simulink library "UXFD_Lib"  (R2016b)
settings: Solver=ode45  StartTime=0.0  StopTime=10.0  RelTol=1e-3  EnableMultiTasking=on
undefined symbols (not defined in the file): BreakpointData, BreakpointData1, BreakpointData2, BreakpointData_One_A, BreakpointData_Two_A, E2E_P01DataIDMode, E2E_P01ReceiverStatusType, EnumClass, iBit, initalValue, No_Runnable_Period, ObB_EidBsgStDerat_C, p_OVERRIDE_MASTER_SWITCH, SlDemoSign, SwitchOff_P, SwitchOn_P, Table, TableData_M, VCCTi33, VSysD_FidVehDerat1_C
libraries: simulink x28, CCMLib x11, UXFD_Lib x8, canmsglib x2, PTCC_Lib x1, hdlsllib x1
(part 6 of 7)

== system UXFD_Lib/Standard/Discrete dynamics/LPF2_omega ==
  u : Inport
  w : Inport  Port=2
  z : Inport  Port=3
  Constant : Constant  Value=2  mask(TL_Constant){data={'output',{'type','Float32'},'date',735300.29222866893}}
      settings: CopyFcn=if exist('tl_reset_reviewflag','file')==2,tl_reset_reviewflag(gcbh);end  DeleteFcn=if exist('delete_tlblock','file')==2,delete_tlblock(gcbh);end  NameChangeFcn=if exist('rename_tlblock','file')==2,rename_tlblock(gcbh);end  OpenFcn=if exist('tl_open_blockdlg','file')==2,tl_open_blockdlg(gcbh);else,open_system(gcbh,'parameter');end
      mask Help: eval(['if exist(''tl_online_help'',''file'') == 2, tl_online_help(''Topic'',''TL_Constant''),else, web([''jar:file:///'',matlabroot,''/help/toolbox/simulink/help.jar!/slref/' lower(get_param(gcbh,'Blocktype')) '.html''], ''-helpbrowser''),end'])
      mask Display: plot([-0.05, 1.05, NaN, -0.05, 1.05],[.01, .01, NaN, .99, .99])
  Constant2 : Constant  Value=2  mask(TL_Constant){data={'output',{'type','Float32'},'date',735300.29222841433}}
      settings: CopyFcn=if exist('tl_reset_reviewflag','file')==2,tl_reset_reviewflag(gcbh);end  DeleteFcn=if exist('delete_tlblock','file')==2,delete_tlblock(gcbh);end  NameChangeFcn=if exist('rename_tlblock','file')==2,rename_tlblock(gcbh);end  OpenFcn=if exist('tl_open_blockdlg','file')==2,tl_open_blockdlg(gcbh);else,open_system(gcbh,'parameter');end
      mask Help: eval(['if exist(''tl_online_help'',''file'') == 2, tl_online_help(''Topic'',''TL_Constant''),else, web([''jar:file:///'',matlabroot,''/help/toolbox/simulink/help.jar!/slref/' lower(get_param(gcbh,'Blocktype')) '.html''], ''-helpbrowser''),end'])
      mask Display: plot([-0.05, 1.05, NaN, -0.05, 1.05],[.01, .01, NaN, .99, .99])
  Constant3 : Constant  mask(TL_Constant){data={'output',{'type','Float32'},'date',735300.29222815973}}
      settings: CopyFcn=if exist('tl_reset_reviewflag','file')==2,tl_reset_reviewflag(gcbh);end  DeleteFcn=if exist('delete_tlblock','file')==2,delete_tlblock(gcbh);end  NameChangeFcn=if exist('rename_tlblock','file')==2,rename_tlblock(gcbh);end  OpenFcn=if exist('tl_open_blockdlg','file')==2,tl_open_blockdlg(gcbh);else,open_system(gcbh,'parameter');end
      mask Help: eval(['if exist(''tl_online_help'',''file'') == 2, tl_online_help(''Topic'',''TL_Constant''),else, web([''jar:file:///'',matlabroot,''/help/toolbox/simulink/help.jar!/slref/' lower(get_param(gcbh,'Blocktype')) '.html''], ''-helpbrowser''),end'])
      mask Display: plot([-0.05, 1.05, NaN, -0.05, 1.05],[.01, .01, NaN, .99, .99])
  Product : Product  Inputs=**  SaturateOnIntegerOverflow=on  RndMeth=Zero  InputSameDT=on  OutDataTypeStr=Inherit: Same as first input  mask(TL_Product){data={'logdata',{'maxnumvals',4096,'plotchannels',[]},'output',{'type','Float32'},'date',735300.29222787032}}
      settings: CopyFcn=if exist('tl_reset_reviewflag','file')==2,tl_reset_reviewflag(gcbh);end  DeleteFcn=if exist('delete_tlblock','file')==2,delete_tlblock(gcbh);end  NameChangeFcn=if exist('rename_tlblock','file')==2,rename_tlblock(gcbh);end  OpenFcn=if exist('tl_open_blockdlg','file')==2,tl_open_blockdlg(gcbh);else,open_system(gcbh,'parameter');end
      mask Help: eval(['if exist(''tl_online_help'',''file'') == 2, tl_online_help(''Topic'',''TL_Product''),else, web([''jar:file:///'',matlabroot,''/help/toolbox/simulink/help.jar!/slref/' lower(get_param(gcbh,'Blocktype')) '.html''], ''-helpbrowser''),end'])
      mask Display: plot([-0.05, 1.05, NaN, -0.05, 1.05],[.01, .01, NaN, .99, .99])
  Product1 : Product  Inputs=***  SaturateOnIntegerOverflow=on  RndMeth=Zero  InputSameDT=on  OutDataTypeStr=Inherit: Same as first input  mask(TL_Product){data={'logdata',{'maxnumvals',4096,'plotchannels',[]},'output',{'type','Float32'},'date',735300.29222759255}}
      settings: CopyFcn=if exist('tl_reset_reviewflag','file')==2,tl_reset_reviewflag(gcbh);end  DeleteFcn=if exist('delete_tlblock','file')==2,delete_tlblock(gcbh);end  NameChangeFcn=if exist('rename_tlblock','file')==2,rename_tlblock(gcbh);end  OpenFcn=if exist('tl_open_blockdlg','file')==2,tl_open_blockdlg(gcbh);else,open_system(gcbh,'parameter');end
      mask Help: eval(['if exist(''tl_online_help'',''file'') == 2, tl_online_help(''Topic'',''TL_Product''),else, web([''jar:file:///'',matlabroot,''/help/toolbox/simulink/help.jar!/slref/' lower(get_param(gcbh,'Blocktype')) '.html''], ''-helpbrowser''),end'])
      mask Display: plot([-0.05, 1.05, NaN, -0.05, 1.05],[.01, .01, NaN, .99, .99])
  Product3 : Product  Inputs=**  SaturateOnIntegerOverflow=on  RndMeth=Zero  InputSameDT=on  OutDataTypeStr=Inherit: Same as first input  mask(TL_Product){data={'logdata',{'maxnumvals',4096,'plotchannels',[]},'output',{'type','Float32'},'date',735300.29222732643}}
      settings: CopyFcn=if exist('tl_reset_reviewflag','file')==2,tl_reset_reviewflag(gcbh);end  DeleteFcn=if exist('delete_tlblock','file')==2,delete_tlblock(gcbh);end  NameChangeFcn=if exist('rename_tlblock','file')==2,rename_tlblock(gcbh);end  OpenFcn=if exist('tl_open_blockdlg','file')==2,tl_open_blockdlg(gcbh);else,open_system(gcbh,'parameter');end
      mask Help: eval(['if exist(''tl_online_help'',''file'') == 2, tl_online_help(''Topic'',''TL_Product''),else, web([''jar:file:///'',matlabroot,''/help/toolbox/simulink/help.jar!/slref/' lower(get_param(gcbh,'Blocktype')) '.html''], ''-helpbrowser''),end'])
      mask Display: plot([-0.05, 1.05, NaN, -0.05, 1.05],[.01, .01, NaN, .99, .99])
  Product4 : Product  Inputs=**  SaturateOnIntegerOverflow=on  RndMeth=Zero  InputSameDT=on  OutDataTypeStr=Inherit: Same as first input  mask(TL_Product){data={'logdata',{'maxnumvals',4096,'plotchannels',[]},'output',{'type','Float32'},'date',735300.29222704866}}
      settings: CopyFcn=if exist('tl_reset_reviewflag','file')==2,tl_reset_reviewflag(gcbh);end  DeleteFcn=if exist('delete_tlblock','file')==2,delete_tlblock(gcbh);end  NameChangeFcn=if exist('rename_tlblock','file')==2,rename_tlblock(gcbh);end  OpenFcn=if exist('tl_open_blockdlg','file')==2,tl_open_blockdlg(gcbh);else,open_system(gcbh,'parameter');end
      mask Help: eval(['if exist(''tl_online_help'',''file'') == 2, tl_online_help(''Topic'',''TL_Product''),else, web([''jar:file:///'',matlabroot,''/help/toolbox/simulink/help.jar!/slref/' lower(get_param(gcbh,'Blocktype')) '.html''], ''-helpbrowser''),end'])
      mask Display: plot([-0.05, 1.05, NaN, -0.05, 1.05],[.01, .01, NaN, .99, .99])
  Product5 : Product  Inputs=*/  SaturateOnIntegerOverflow=on  RndMeth=Zero  InputSameDT=on  OutDataTypeStr=Inherit: Same as first input  mask(TL_Product){data={'logdata',{'maxnumvals',4096,'plotchannels',[]},'output',{'type','Float32'},'date',735300.29222677078}}
      settings: CopyFcn=if exist('tl_reset_reviewflag','file')==2,tl_reset_reviewflag(gcbh);end  DeleteFcn=if exist('delete_tlblock','file')==2,delete_tlblock(gcbh);end  NameChangeFcn=if exist('rename_tlblock','file')==2,rename_tlblock(gcbh);end  OpenFcn=if exist('tl_open_blockdlg','file')==2,tl_open_blockdlg(gcbh);else,open_system(gcbh,'parameter');end
      mask Help: eval(['if exist(''tl_online_help'',''file'') == 2, tl_online_help(''Topic'',''TL_Product''),else, web([''jar:file:///'',matlabroot,''/help/toolbox/simulink/help.jar!/slref/' lower(get_param(gcbh,'Blocktype')) '.html''], ''-helpbrowser''),end'])
      mask Display: plot([-0.05, 1.05, NaN, -0.05, 1.05],[.01, .01, NaN, .99, .99])
  Product6 : Product  Inputs=**  SaturateOnIntegerOverflow=on  RndMeth=Zero  InputSameDT=on  OutDataTypeStr=Inherit: Same as first input  mask(TL_Product){data={'logdata',{'maxnumvals',4096,'plotchannels',[]},'output',{'type','Float32'},'date',735300.29222649301}}
      settings: CopyFcn=if exist('tl_reset_reviewflag','file')==2,tl_reset_reviewflag(gcbh);end  DeleteFcn=if exist('delete_tlblock','file')==2,delete_tlblock(gcbh);end  NameChangeFcn=if exist('rename_tlblock','file')==2,rename_tlblock(gcbh);end  OpenFcn=if exist('tl_open_blockdlg','file')==2,tl_open_blockdlg(gcbh);else,open_system(gcbh,'parameter');end
      mask Help: eval(['if exist(''tl_online_help'',''file'') == 2, tl_online_help(''Topic'',''TL_Product''),else, web([''jar:file:///'',matlabroot,''/help/toolbox/simulink/help.jar!/slref/' lower(get_param(gcbh,'Blocktype')) '.html''], ''-helpbrowser''),end'])
      mask Display: plot([-0.05, 1.05, NaN, -0.05, 1.05],[.01, .01, NaN, .99, .99])
  Sum1 : Sum  Inputs=+--  SaturateOnIntegerOverflow=on  InputSameDT=on  OutDataTypeStr=Inherit: Same as first input  mask(TL_Sum){data={'logdata',{'maxnumvals',4096,'plotchannels',[]},'output',{'type','Float32'},'date',735300.29222619208}}
      settings: CopyFcn=if exist('tl_reset_reviewflag','file')==2,tl_reset_reviewflag(gcbh);end  DeleteFcn=if exist('delete_tlblock','file')==2,delete_tlblock(gcbh);end  NameChangeFcn=if exist('rename_tlblock','file')==2,rename_tlblock(gcbh);end  OpenFcn=if exist('tl_open_blockdlg','file')==2,tl_open_blockdlg(gcbh);else,open_system(gcbh,'parameter');end
      mask Help: eval(['if exist(''tl_online_help'',''file'') == 2, tl_online_help(''Topic'',''TL_Sum''),else, web([''jar:file:///'',matlabroot,''/help/toolbox/simulink/help.jar!/slref/' lower(get_param(gcbh,'Blocktype')) '.html''], ''-helpbrowser''),end'])
      mask Display: plot([-0.05, 1.05, NaN, -0.05, 1.05],[.01, .01, NaN, .99, .99])
  Sum2 : Sum  Inputs=--  SaturateOnIntegerOverflow=on  InputSameDT=on  OutDataTypeStr=Inherit: Same as first input  mask(TL_Sum){data={'logdata',{'maxnumvals',4096,'plotchannels',[]},'output',{'type','Float32'},'date',735300.29222592595}}
      settings: CopyFcn=if exist('tl_reset_reviewflag','file')==2,tl_reset_reviewflag(gcbh);end  DeleteFcn=if exist('delete_tlblock','file')==2,delete_tlblock(gcbh);end  NameChangeFcn=if exist('rename_tlblock','file')==2,rename_tlblock(gcbh);end  OpenFcn=if exist('tl_open_blockdlg','file')==2,tl_open_blockdlg(gcbh);else,open_system(gcbh,'parameter');end
      mask Help: eval(['if exist(''tl_online_help'',''file'') == 2, tl_online_help(''Topic'',''TL_Sum''),else, web([''jar:file:///'',matlabroot,''/help/toolbox/simulink/help.jar!/slref/' lower(get_param(gcbh,'Blocktype')) '.html''], ''-helpbrowser''),end'])
      mask Display: plot([-0.05, 1.05, NaN, -0.05, 1.05],[.01, .01, NaN, .99, .99])
  Sum3 : Sum  Inputs=+++  SaturateOnIntegerOverflow=on  InputSameDT=on  OutDataTypeStr=Inherit: Same as first input  mask(TL_Sum){data={'logdata',{'maxnumvals',4096,'plotchannels',[]},'output',{'type','Float32'},'date',735300.29222564818}}
      settings: CopyFcn=if exist('tl_reset_reviewflag','file')==2,tl_reset_reviewflag(gcbh);end  DeleteFcn=if exist('delete_tlblock','file')==2,delete_tlblock(gcbh);end  NameChangeFcn=if exist('rename_tlblock','file')==2,rename_tlblock(gcbh);end  OpenFcn=if exist('tl_open_blockdlg','file')==2,tl_open_blockdlg(gcbh);else,open_system(gcbh,'parameter');end
      mask Help: eval(['if exist(''tl_online_help'',''file'') == 2, tl_online_help(''Topic'',''TL_Sum''),else, web([''jar:file:///'',matlabroot,''/help/toolbox/simulink/help.jar!/slref/' lower(get_param(gcbh,'Blocktype')) '.html''], ''-helpbrowser''),end'])
      mask Display: plot([-0.05, 1.05, NaN, -0.05, 1.05],[.01, .01, NaN, .99, .99])
  UnitDelay1 : UnitDelay  SampleTime=-1  mask(TL_UnitDelay){data={'logdata',{'maxnumvals',4096,'plotchannels',[]},'output',{'type','Float32'},'state',{'type','Float32'},'date',735300.29222532408}}
      settings: CopyFcn=if exist('tl_reset_reviewflag','file')==2,tl_reset_reviewflag(gcbh);end  DeleteFcn=if exist('delete_tlblock','file')==2,delete_tlblock(gcbh);end  NameChangeFcn=if exist('rename_tlblock','file')==2,rename_tlblock(gcbh);end  OpenFcn=if exist('tl_open_blockdlg','file')==2,tl_open_blockdlg(gcbh);else,open_system(gcbh,'parameter');end
      mask Help: eval(['if exist(''tl_online_help'',''file'') == 2, tl_online_help(''Topic'',''TL_UnitDelay''),else, web([''jar:file:///'',matlabroot,''/help/toolbox/simulink/help.jar!/slref/' lower(get_param(gcbh,'Blocktype')) '.html''], ''-helpbrowser''),end'])
      mask Display: plot([-0.05, 1.05, NaN, -0.05, 1.05],[.01, .01, NaN, .99, .99])
  UnitDelay3 : UnitDelay  SampleTime=-1  mask(TL_UnitDelay){data={'logdata',{'maxnumvals',4096,'plotchannels',[]},'output',{'type','Float32'},'state',{'type','Float32'},'date',735300.29222478007}}
      settings: CopyFcn=if exist('tl_reset_reviewflag','file')==2,tl_reset_reviewflag(gcbh);end  DeleteFcn=if exist('delete_tlblock','file')==2,delete_tlblock(gcbh);end  NameChangeFcn=if exist('rename_tlblock','file')==2,rename_tlblock(gcbh);end  OpenFcn=if exist('tl_open_blockdlg','file')==2,tl_open_blockdlg(gcbh);else,open_system(gcbh,'parameter');end
      mask Help: eval(['if exist(''tl_online_help'',''file'') == 2, tl_online_help(''Topic'',''TL_UnitDelay''),else, web([''jar:file:///'',matlabroot,''/help/toolbox/simulink/help.jar!/slref/' lower(get_param(gcbh,'Blocktype')) '.html''], ''-helpbrowser''),end'])
      mask Display: plot([-0.05, 1.05, NaN, -0.05, 1.05],[.01, .01, NaN, .99, .99])
  ts : DataStoreRead  DataStoreName=ts  mask(TL_DataStoreRead){data={'logdata',{'plotchannels',[]},'date',735300.29222303245}}
      settings: AttributesFormatString=ts  DeleteFcn=if exist('delete_tlblock','file')==2,delete_tlblock(gcbh);end  NameChangeFcn=if exist('rename_tlblock','file')==2,rename_tlblock(gcbh);end  OpenFcn=if exist('tl_open_blockdlg','file')==2,tl_open_blockdlg(gcbh);else,open_system(gcbh,'parameter');end
      mask Help: eval(['if exist(''tl_online_help'',''file'') == 2, tl_online_help(''Topic'',''TL_DataStoreRead''),else, web([''jar:file:///'',matlabroot,''/help/toolbox/simulink/help.jar!/slref/' lower(get_param(gcbh,'Blocktype')) '.html''], ''-helpbrowser''),end'])
      mask Display: plot([-0.05, 1.05, NaN, -0.05, 1.05],[.01, .01, NaN, .99, .99])
  y : Outport
  wires:
  z/1 -> Product1/2
  UnitDelay3/1 -> Sum1/3
  Product3/1 -> Product6/2, Sum3/2
  Sum3/1 -> Product5/2
  Constant3/1 -> Sum3/3
  Product5/1 -> y/1, UnitDelay1/1
  Constant2/1 -> Sum2/1
  u/1 -> Product6/1
  Product6/1 -> Sum1/1
  Product4/1 -> Sum1/2
  Sum1/1 -> Product5/1
  Sum2/1 -> Product4/1
  ts/1 -> Product/2
  w/1 -> Product/1
  Constant/1 -> Product1/3
  Product1/1 -> Sum3/1, Sum2/2
  UnitDelay1/1 -> Product4/2, UnitDelay3/1
  Product/1 -> Product1/1, Product3/2, Product3/1

== system UXFD_Lib/Standard/Discrete dynamics/RateLimit ==
  u : Inport
  d : Inport  Port=2
  Add : Sum  Inputs=+-
  Add1 : Sum
  MinMax : MinMax  Function=max  Inputs=2
  MinMax1 : MinMax  Inputs=2
  Product : Product
  Product1 : Product
  Unit Delay : UnitDelay  SampleTime=-1
  ts : DataStoreRead  DataStoreName=ts
  y : Outport
  wires:
  d/1 -> Product/1, Product1/2
  Product/1 -> Add1/1
  ts/1 -> Product/2, Product1/1
  Product1/1 -> Add/2
  Add/1 -> MinMax/2
  MinMax/1 -> MinMax1/1
  Unit Delay/1 -> Add1/2, Add/1
  Add1/1 -> MinMax1/2
  u/1 -> MinMax/1
  MinMax1/1 -> y/1, Unit Delay/1

== system UXFD_Lib/Standard/Discrete dynamics/RateLimit1 ==
  In1 : Inport
  r : Inport  Port=2
  dr : Inport  Port=3
  r1 : Inport  Port=4
  Abs : Abs
  Add : Sum  Inputs=+-
  Add1 : Sum
  MinMax : MinMax  Function=max  Inputs=2
  MinMax1 : MinMax  Inputs=2
  Product : Product
  Product1 : Product
  Switch : Switch  Criteria=u2 > Threshold
  Unit Delay : UnitDelay  SampleTime=-1
  ts : DataStoreRead  DataStoreName=ts
  y : Outport
  wires:
  Abs/1 -> Add/2
  In1/1 -> Switch/1, MinMax/1
  Add1/1 -> MinMax1/2
  Unit Delay/1 -> Add1/2, Add/1
  MinMax/1 -> MinMax1/1
  Product1/1 -> Abs/1
  ts/1 -> Product1/1, Product/2
  Product/1 -> Add1/1
  dr/1 -> Product/1
  MinMax1/1 -> Switch/3
  r/1 -> Switch/2
  Switch/1 -> y/1, Unit Delay/1
  r1/1 -> Product1/2
  Add/1 -> MinMax/2

== system UXFD_Lib/Standard/Discrete dynamics/xbackground1 ==

== system UXFD_Lib/Standard/Discrete dynamics/xbackground2 ==

== system UXFD_Lib/Standard/Discrete dynamics/xbackground3 ==

== system UXFD_Lib/Standard/Discrete dynamics/xbackground4 ==

== system UXFD_Lib/Standard/Discrete dynamics/xbackground5 ==

== system UXFD_Lib/Standard/Discrete dynamics/xbackground6 ==

== system UXFD_Lib/Standard/Discrete dynamics/xbackground7 ==

== system UXFD_Lib/Standard/Math/AbsForBoschCompiler ==
  In1 : Inport
  Gain : Gain  Gain=-1  OutDataTypeStr=Inherit: Same as input  ParamDataTypeStr=Inherit: Same as input  mask(TL_Gain){data={'logdata',{'plotchannels',[]},'output',{'type','Float32','unit','-'},'date',735300.29225025466}}
      settings: CopyFcn=if exist('tl_reset_reviewflag','file')==2,tl_reset_reviewflag(gcbh);end  DeleteFcn=if exist('delete_tlblock','file')==2,delete_tlblock(gcbh);end  NameChangeFcn=if exist('rename_tlblock','file')==2,rename_tlblock(gcbh);end  OpenFcn=if exist('tl_open_blockdlg','file')==2,tl_open_blockdlg(gcbh);else,open_system(gcbh,'parameter');end
      mask Help: eval(['if exist(''tl_online_help'',''file'') == 2, tl_online_help(''Topic'',''TL_Gain''),else, web([''jar:file:///'',matlabroot,''/help/toolbox/simulink/help.jar!/slref/' lower(get_param(gcbh,'Blocktype')) '.html''], ''-helpbrowser''),end'])
      mask Display: plot([0, .9, 0],[.05, .5, .95])
  Switch1 : Switch  mask(TL_Switch){data={'logdata',{'plotchannels',[]},'output',{'name','r$N_$L','class','CVC_DISP32','type','Float32'},'date',737070.42928155093}}
      settings: CopyFcn=if exist('tl_reset_reviewflag','file')==2,tl_reset_reviewflag(gcbh);end  DeleteFcn=if exist('delete_tlblock','file')==2,delete_tlblock(gcbh);end  NameChangeFcn=if exist('rename_tlblock','file')==2,rename_tlblock(gcbh);end  OpenFcn=if exist('tl_open_blockdlg','file')==2,tl_open_blockdlg(gcbh);else,open_system(gcbh,'parameter');end
      mask Help: eval(['if exist(''tl_online_help'',''file'') == 2, tl_online_help(''Topic'',''TL_Switch''),else, web([''jar:file:///'',matlabroot,''/help/toolbox/simulink/help.jar!/slref/' lower(get_param(gcbh,'Blocktype')) '.html''], ''-helpbrowser''),end'])
      mask Display: plot([-0.05, 1.05, NaN, -0.05, 1.05],[.01, .01, NaN, .99, .99])
  Out1 : Outport
  wires:
  Gain/1 -> Switch1/3
  In1/1 -> Gain/1, Switch1/2, Switch1/1
  Switch1/1 -> Out1/1  "rt_DFT2RevArgAbs"

== system UXFD_Lib/Standard/Math/Floor ==
  In1 : Inport
  Add : Sum  Inputs=+-
  Constant : Constant
  mod1 : Subsystem  mask(GL_Mod_1.0){}
      mask help: Signed remainder after division.
      mask Display: disp('mod')
  Out1 : Outport
  wires:
  Constant/1 -> mod1/2(In2)
  Add/1 -> Out1/1
  In1/1 -> mod1/1(In1), Add/1
  mod1/1(Out1) -> Add/2

== system UXFD_Lib/Standard/Math/Interpolation ==
  In1 : Inport
  x1 : Inport  Port=2
  y1 : Inport  Port=3
  x2 : Inport  Port=4
  y2 : Inport  Port=5
  Add : Sum  Inputs=+-
  Add1 : Sum  Inputs=+-
  Add2 : Sum  Inputs=+-
  Add3 : Sum
  Constant : Constant
  One3 : Constant  Value=1e-6  OutDataTypeStr=single  mask(TL_Constant){data={'output',{'type','Float32'},'date',735300.29224869213}}
      settings: CopyFcn=if exist('tl_reset_reviewflag','file')==2,tl_reset_reviewflag(gcbh);end  DeleteFcn=if exist('delete_tlblock','file')==2,delete_tlblock(gcbh);end  NameChangeFcn=if exist('rename_tlblock','file')==2,rename_tlblock(gcbh);end  OpenFcn=if exist('tl_open_blockdlg','file')==2,tl_open_blockdlg(gcbh);else,open_system(gcbh,'parameter');end
      mask Help: eval(['if exist(''tl_online_help'',''file'') == 2, tl_online_help(''Topic'',''TL_Constant''),else, web([''jar:file:///'',matlabroot,''/help/toolbox/simulink/help.jar!/slref/' lower(get_param(gcbh,'Blocktype')) '.html''], ''-helpbrowser''),end'])
      mask Display: plot([-0.05, 1.05, NaN, -0.05, 1.05],[.01, .01, NaN, .99, .99])
  Product : Product
  Product1 : Product
  Safe_Divide : Subsystem  mask(GL_SafeDivide_1.0){}
      mask help:
      | Safe Divide, prevents division by zero.
      |
      | if abs(denominator) > eps then
      |     output = numerator / denominator
      | else
      |     output = numerator / eps
      |
      | Attention!
      | Use this block only when there is a risk for division by zero.
      mask init:
      | set_param(gcb,'LinkStatus','none');
      mask Display:
      | port_label('input', 1, 'x')
      | port_label('input', 2, '÷')
      | port_label('input', 3, 'eps')
  Out1 : Outport
  wires:
  In1/1 -> Add/1
  x1/1 -> Add1/2, Add/2
  Add/1 -> Safe_Divide/1(In3)
  Constant/1 -> Add2/1
  Add2/1 -> Product/2
  Product1/1 -> Add3/2
  Product/1 -> Add3/1
  Add1/1 -> Safe_Divide/2(In2)
  Add3/1 -> Out1/1
  y1/1 -> Product/1
  y2/1 -> Product1/2
  Safe_Divide/1(Out1) -> Product1/1, Add2/2
  x2/1 -> Add1/1
  One3/1 -> Safe_Divide/3(In1)

== system UXFD_Lib/Standard/Math/LimitInterpolation ==
  In1 : Inport
  x1 : Inport  Port=2
  y1 : Inport  Port=3
  x2 : Inport  Port=4
  y2 : Inport  Port=5
  Add : Sum  Inputs=+-
  Add1 : Sum  Inputs=+-
  Add2 : Sum  Inputs=+-
  Add3 : Sum
  Constant : Constant
  Constant1 : Constant  Value=0
  Constant2 : Constant
  One3 : Constant  Value=1e-6  OutDataTypeStr=single  mask(TL_Constant){data={'output',{'type','Float32'},'date',735300.29224403936}}
      settings: CopyFcn=if exist('tl_reset_reviewflag','file')==2,tl_reset_reviewflag(gcbh);end  DeleteFcn=if exist('delete_tlblock','file')==2,delete_tlblock(gcbh);end  NameChangeFcn=if exist('rename_tlblock','file')==2,rename_tlblock(gcbh);end  OpenFcn=if exist('tl_open_blockdlg','file')==2,tl_open_blockdlg(gcbh);else,open_system(gcbh,'parameter');end
      mask Help: eval(['if exist(''tl_online_help'',''file'') == 2, tl_online_help(''Topic'',''TL_Constant''),else, web([''jar:file:///'',matlabroot,''/help/toolbox/simulink/help.jar!/slref/' lower(get_param(gcbh,'Blocktype')) '.html''], ''-helpbrowser''),end'])
      mask Display: plot([-0.05, 1.05, NaN, -0.05, 1.05],[.01, .01, NaN, .99, .99])
  Product : Product
  Product1 : Product
  Safe_Divide : Subsystem  mask(GL_SafeDivide_1.0){}
      mask help:
      | Safe Divide, prevents division by zero.
      |
      | if abs(denominator) > eps then
      |     output = numerator / denominator
      | else
      |     output = numerator / eps
      |
      | Attention!
      | Use this block only when there is a risk for division by zero.
      mask init:
      | set_param(gcb,'LinkStatus','none');
      mask Display:
      | port_label('input', 1, 'x')
      | port_label('input', 2, '÷')
      | port_label('input', 3, 'eps')
  Saturation : Subsystem  mask(GL_Saturation_1.0){}
      mask help:
      | If input_1 > input_2
      |   output = input_2
      | elseif input_1 < input_3
      |   output = input_3
      | else
      |   output = input_1
      |
      | Note that if the lower limit is set above the upper limit, the output will take the value of the input to the lower limit port.
      mask init:
      | set_param(gcb,'LinkStatus','none');
      mask Display: plot([0.3, 0.5, 0.7, 0.9], [0, 0, 1, 1])
  Out1 : Outport
  wires:
  x2/1 -> Add1/1
  Safe_Divide/1(Out1) -> Saturation/1(u)
  y2/1 -> Product1/2
  y1/1 -> Product/1
  Add3/1 -> Out1/1
  Add1/1 -> Safe_Divide/2(In2)
  Product/1 -> Add3/1
  Product1/1 -> Add3/2
  Add2/1 -> Product/2
  Saturation/1(y) -> Product1/1, Add2/2
  Constant2/1 -> Add2/1
  Constant1/1 -> Saturation/3(L)
  Constant/1 -> Saturation/2(U)
  Add/1 -> Safe_Divide/1(In3)
  x1/1 -> Add1/2, Add/2
  In1/1 -> Add/1
  One3/1 -> Safe_Divide/3(In1)

== system UXFD_Lib/Standard/Math/Round ==
  In1 : Inport
  Add : Sum
  Add1 : Sum  Inputs=+-
  Constant : Constant  Value=0.5
  Constant1 : Constant
  mod : Subsystem  mask(PAG_mod_LV1.5_BV1){}
      mask help: Signed remainder after division.
      mask Display: disp('mod')
  Out1 : Outport
  wires:
  mod/1(Out1) -> Add1/2
  In1/1 -> Add/1
  Add/1 -> Add1/1, mod/1(In1)
  Add1/1 -> Out1/1
  Constant1/1 -> mod/2(In2)
  Constant/1 -> Add/2

== system UXFD_Lib/Standard/Math/Safe_Divide ==
  In2 : Inport
  In1 : Inport  Port=2
  In3 : Inport  Port=3
  Constant : Constant  Value=0  OutDataTypeStr=Inherit: Inherit via back propagation
  Gain : Gain  Gain=-1
  LogicalSwitch : Subsystem  mask(PAG_Switch_LV1.6_BV2){}
      mask help:
      | Pass through input 1 when input 3 is true;
      | otherwise, pass through input 2
      mask Display:
      | plot([-0.1 0.2 0.2], [0.85 0.85 0.75])
      | plot([-0.1 0.2 0.2], [0.5 0.5 0.6])
      | plot([0.8 1.1], [0.5 0.5])
      | plot([0.15 0.8], [0.6 0.5])
      | plot([-0.1 0.5 0.5], [0.15 0.15 0.6])
  Max : MinMax  Function=max  Inputs=2
  MinMax1 : MinMax  Inputs=2
  Product1 : Product  Inputs=*/
  Relational Operator : RelationalOperator  Operator=<  OutDataTypeStr=boolean  RndMeth=Nearest
  Out1 : Outport
  wires:
  Relational Operator/1 -> LogicalSwitch/3(In3)
  Gain/1 -> MinMax1/2
  Product1/1 -> Out1/1
  Constant/1 -> Relational Operator/2
  In2/1 -> Product1/1
  LogicalSwitch/1(Out1) -> Product1/2
  Max/1 -> LogicalSwitch/2(In2)
  MinMax1/1 -> LogicalSwitch/1(In1)
  In3/1 -> Max/1, Gain/1
  In1/1 -> MinMax1/1, Max/2, Relational Operator/1

== system UXFD_Lib/Standard/Math/Saturation ==
  u : Inport
  U : Inport  Port=2
  L : Inport  Port=3
  MinMax : MinMax  Inputs=2
  MinMax1 : MinMax  Function=max  Inputs=2
  y : Outport
  wires:
  MinMax/1 -> MinMax1/1
  U/1 -> MinMax/1
  u/1 -> MinMax/2
  MinMax1/1 -> y/1
  L/1 -> MinMax1/2

== system UXFD_Lib/Standard/Math/mod ==
  In1 : Inport
  In2 : Inport  Port=2
  Mod : Math  Operator=mod  SaturateOnIntegerOverflow=on
  Out1 : Outport
  wires:
  In1/1 -> Mod/1
  Mod/1 -> Out1/1
  In2/1 -> Mod/2

== system UXFD_Lib/Standard/Math/rem ==
  In1 : Inport
  In2 : Inport  Port=2
  rem : Math  Operator=rem  SaturateOnIntegerOverflow=on
  Out1 : Outport
  wires:
  In1/1 -> rem/1
  rem/1 -> Out1/1
  In2/1 -> rem/2

== system UXFD_Lib/Standard/Math/sign_real ==
  In1 : Inport
  Constant : Constant  Value=-1
      settings: CopyFcn=set_param(gcbh,'ShowName','off');
  Constant1 : Constant
      settings: CopyFcn=set_param(gcbh,'ShowName','off');
  Constant2 : Constant  Value=0
      settings: CopyFcn=set_param(gcbh,'ShowName','off');
  Constant3 : Constant  Value=0
      settings: CopyFcn=set_param(gcbh,'ShowName','off');
  Constant4 : Constant  Value=0
      settings: CopyFcn=set_param(gcbh,'ShowName','off');
  Relational Operator : RelationalOperator  Operator===  OutDataTypeStr=boolean  RndMeth=Nearest
  Relational Operator1 : RelationalOperator  Operator=>  OutDataTypeStr=boolean  RndMeth=Nearest
  Switch : Switch  Criteria=u2 ~= 0  OutDataTypeStr=Inherit: Inherit via back propagation  RndMeth=Round  SaturateOnIntegerOverflow=on  InputSameDT=on
      mask init:
      | set_param(gcb,'LinkStatus','none');
      settings: CopyFcn=set_param(gcb,'showname','off');
      mask Display:
      | plot([0.54 0.65],[0.92 0.92])
      | plot([0.6 0.6],[0.84 0.92])
      | 
      | plot([0.54 0.54],[0.01 0.14])
      | plot([0.54 0.65],[0.14 0.14])
      | plot([0.54 0.625],[0.08 0.08])
  Switch1 : Switch  Criteria=u2 ~= 0  OutDataTypeStr=Inherit: Inherit via back propagation  RndMeth=Round  SaturateOnIntegerOverflow=on  InputSameDT=on
      mask init:
      | set_param(gcb,'LinkStatus','none');
      settings: CopyFcn=set_param(gcb,'showname','off');
      mask Display:
      | plot([0.54 0.65],[0.92 0.92])
      | plot([0.6 0.6],[0.84 0.92])
      | 
      | plot([0.54 0.54],[0.02 0.14])
      | plot([0.54 0.65],[0.14 0.14])
      | plot([0.54 0.625],[0.08 0.08])
  Out1 : Outport
  wires:
  Relational Operator/1 -> Switch1/2
  Relational Operator1/1 -> Switch/2
  Switch/1 -> Switch1/3
  Constant/1 -> Switch/3
  Constant1/1 -> Switch/1
  Constant2/1 -> Switch1/1
  Constant3/1 -> Relational Operator/2
  Constant4/1 -> Relational Operator1/2
  In1/1 -> Relational Operator1/1, Relational Operator/1
  Switch1/1 -> Out1/1

== system UXFD_Lib/Standard/Math/xbackground1 ==

== system UXFD_Lib/Standard/Math/xbackground10 ==

== system UXFD_Lib/Standard/Math/xbackground2 ==

== system UXFD_Lib/Standard/Math/xbackground3 ==

== system UXFD_Lib/Standard/Relation&Logic/ConditionArbitration ==
  Condition1 : Inport  OutDataTypeStr=boolean
  Condition2 : Inport  Port=2  OutDataTypeStr=boolean
  Val_0_0 : Inport  Port=3
  Val_0_1 : Inport  Port=4
  Val_1_0 : Inport  Port=5
  Val_1_1 : Inport  Port=6
  Data Type Conversion : DataTypeConversion  RndMeth=Simplest  SaturateOnIntegerOverflow=on
  Switch : Switch  Criteria=u2 ~= 0  OutDataTypeStr=Inherit: Inherit via back propagation  RndMeth=Simplest  SaturateOnIntegerOverflow=on  InputSameDT=on
      mask init:
      | set_param(gcb, 'LinkStatus', 'none');
      mask Display:
      | plot([0.54 0.65],[0.92 0.92])
      | plot([0.6 0.6],[0.84 0.92])
      | 
      | plot([0.54 0.54],[0.05 0.14])
      | plot([0.54 0.65],[0.14 0.14])
      | plot([0.54 0.625],[0.08 0.08])
  Switch1 : Switch  Criteria=u2 ~= 0  OutDataTypeStr=Inherit: Inherit via back propagation  RndMeth=Simplest  SaturateOnIntegerOverflow=on  InputSameDT=on
      mask init:
      | set_param(gcb, 'LinkStatus', 'none');
      mask Display:
      | plot([0.54 0.65],[0.92 0.92])
      | plot([0.6 0.6],[0.84 0.92])
      | 
      | plot([0.54 0.54],[0.05 0.14])
      | plot([0.54 0.65],[0.14 0.14])
      | plot([0.54 0.625],[0.08 0.08])
  Switch2 : Switch  Criteria=u2 ~= 0  OutDataTypeStr=Inherit: Inherit via back propagation  RndMeth=Simplest  SaturateOnIntegerOverflow=on  InputSameDT=on
      mask init:
      | set_param(gcb, 'LinkStatus', 'none');
      mask Display:
      | plot([0.54 0.65],[0.92 0.92])
      | plot([0.6 0.6],[0.84 0.92])
      | 
      | plot([0.54 0.54],[0.05 0.14])
      | plot([0.54 0.65],[0.14 0.14])
      | plot([0.54 0.625],[0.08 0.08])
  out : Outport
  wires:
  Data Type Conversion/1 -> out/1
  Switch1/1 -> Data Type Conversion/1
  Switch2/1 -> Switch1/3
  Val_0_1/1 -> Switch2/1
  Val_0_0/1 -> Switch2/3
  Val_1_0/1 -> Switch/3
  Switch/1 -> Switch1/1
  Val_1_1/1 -> Switch/1
  Condition1/1 -> Switch1/2
  Condition2/1 -> Switch/2, Switch2/2

== system UXFD_Lib/Standard/Relation&Logic/CounterReset_dec ==
  e : Inport
  r : Inport  Port=2
  rv : Inport  Port=3
  dec : Inport  Port=4
  Add : Sum  Inputs=-+
  Constant : Constant  Value=0
  Constant1 : Constant  Value=0
  MinMax : MinMax  Function=max  Inputs=2
  Switch : Switch  Criteria=u2 ~= 0  Threshold=0.5
  Switch1 : Switch  Criteria=u2 ~= 0  Threshold=0.5
  Unit Delay : UnitDelay  SampleTime=-1
  y : Outport
  wires:
  Switch1/1 -> Add/1
  Constant1/1 -> Switch1/3
  dec/1 -> Switch1/1
  e/1 -> Switch1/2
  r/1 -> Switch/2
  Add/1 -> Switch/3
  rv/1 -> Switch/1
  Switch/1 -> MinMax/2
  Constant/1 -> MinMax/1
  MinMax/1 -> Unit Delay/1, y/1
  Unit Delay/1 -> Add/2

== system UXFD_Lib/Standard/Relation&Logic/CounterReset_uint8 ==
  r : Inport
  rv : Inport  Port=2
  inc : Inport  Port=3
  Add : Sum  SaturateOnIntegerOverflow=on
  Switch1 : Switch  Criteria=u2 ~= 0  OutDataTypeStr=Inherit: Inherit via back propagation  RndMeth=Round  SaturateOnIntegerOverflow=on  InputSameDT=on
      mask init:
      | set_param(gcb,'LinkStatus','none');
      | % 这句的使用场景：
      | % 当模型没有这句时，模型传递给没有模型库的人员会出现红色的错误框
      | % 没有模型库的使用者不能查看此模块
      settings: CopyFcn=set_param(gcb,'showname','off');
      mask Display:
      | plot([0.54 0.65],[0.92 0.92])
      | plot([0.6 0.6],[0.84 0.92])
      | 
      | plot([0.54 0.54],[0.02 0.14])
      | plot([0.54 0.65],[0.14 0.14])
      | plot([0.54 0.625],[0.08 0.08])
  Unit Delay : UnitDelay  SampleTime=-1
  y : Outport
  wires:
  r/1 -> Switch1/2
  Add/1 -> Switch1/3
  rv/1 -> Switch1/1
  Unit Delay/1 -> Add/2
  inc/1 -> Add/1
  Switch1/1 -> y/1, Unit Delay/1

== system UXFD_Lib/Standard/Relation&Logic/CounterReset_uint8_enable ==
  e : Inport
  r : Inport  Port=2
  rv : Inport  Port=3
  inc : Inport  Port=4
  Add : Sum  SaturateOnIntegerOverflow=on
  Constant1 : Constant  Value=0
  Switch : Switch  Criteria=u2 ~= 0  OutDataTypeStr=Inherit: Inherit via back propagation  RndMeth=Round  SaturateOnIntegerOverflow=on  InputSameDT=on
      mask init:
      | set_param(gcb,'LinkStatus','none');
      settings: CopyFcn=set_param(gcb,'showname','off');
      mask Display:
      | plot([0.54 0.65],[0.92 0.92])
      | plot([0.6 0.6],[0.84 0.92])
      | 
      | plot([0.54 0.54],[0.02 0.14])
      | plot([0.54 0.65],[0.14 0.14])
      | plot([0.54 0.625],[0.08 0.08])
  Switch1 : Switch  Criteria=u2 ~= 0  Threshold=0.5
  Unit Delay : UnitDelay  SampleTime=-1
  y : Outport
  wires:
  Unit Delay/1 -> Add/2
  rv/1 -> Switch/1
  Add/1 -> Switch/3
  r/1 -> Switch/2
  e/1 -> Switch1/2
  inc/1 -> Switch1/1
  Switch1/1 -> Add/1
  Constant1/1 -> Switch1/3
  Switch/1 -> y/1, Unit Delay/1

== system UXFD_Lib/Standard/Relation&Logic/EdgeBi ==
  u : Inport
  AND : Logic  Operator=XOR  AllPortsSameDT=off  OutDataTypeStr=boolean
  Unit Delay : UnitDelay  SampleTime=-1
  y : Outport
  wires:
  AND/1 -> y/1
  Unit Delay/1 -> AND/2
  u/1 -> AND/1, Unit Delay/1

== system UXFD_Lib/Standard/Relation&Logic/EdgeFalling ==
  In1 : Inport
  AND : Logic  Operator=NOT  Inputs=1  AllPortsSameDT=off  OutDataTypeStr=boolean
  AND1 : Logic  AllPortsSameDT=off  OutDataTypeStr=boolean
  Unit Delay : UnitDelay  SampleTime=-1
  Out1 : Outport
  wires:
  In1/1 -> AND/1, Unit Delay/1
  AND1/1 -> Out1/1
  Unit Delay/1 -> AND1/2
  AND/1 -> AND1/1

== system UXFD_Lib/Standard/Relation&Logic/EdgeRising ==
  u : Inport
  AND : Logic  Operator=NOT  Inputs=1  AllPortsSameDT=off  OutDataTypeStr=boolean
  AND1 : Logic  AllPortsSameDT=off  OutDataTypeStr=boolean
  Unit Delay : UnitDelay  SampleTime=-1
  y : Outport
  wires:
  u/1 -> Unit Delay/1, AND1/1
  AND1/1 -> y/1
  Unit Delay/1 -> AND/1
  AND/1 -> AND1/2

== system UXFD_Lib/Standard/Relation&Logic/If Action Subsystem ==
  In1 : Inport
  Action Port : ActionPort
  Out1 : Outport
  wires:
  In1/1 -> Out1/1

== system UXFD_Lib/Standard/Relation&Logic/If-Then-Else ==
  If : Inport
  Then : Inport  Port=2
  Else : Inport  Port=3
  Switch : Switch  Criteria=u2 ~= 0  InputSameDT=on
      settings: AttributesFormatString=Require same data type on all input ports = %<InputSameDT>
  Out : Outport
  wires:
  Else/1 -> Switch/3
  Then/1 -> Switch/1
  If/1 -> Switch/2
  Switch/1 -> Out/1

== system UXFD_Lib/Standard/Relation&Logic/RS_FF ==
  S : Inport
  R : Inport  Port=2
  AND : Logic  Operator=NOT  Inputs=1  AllPortsSameDT=off  OutDataTypeStr=boolean
  AND1 : Logic  AllPortsSameDT=off  OutDataTypeStr=boolean
  AND2 : Logic  Operator=OR  AllPortsSameDT=off  OutDataTypeStr=boolean
  Unit Delay : UnitDelay  SampleTime=-1
  Q : Outport
  wires:
  AND/1 -> AND1/1
  R/1 -> AND/1
  S/1 -> AND2/1
  AND2/1 -> AND1/2
  Unit Delay/1 -> AND2/2
  AND1/1 -> Q/1, Unit Delay/1

== system UXFD_Lib/Standard/Relation&Logic/Relay ==
  In2 : Inport
  on : Inport  Port=2
  off : Inport  Port=3
  AND : Logic  Operator=NOT  Inputs=1  AllPortsSameDT=off  OutDataTypeStr=boolean
  AND1 : Logic  Operator=NOT  Inputs=1  AllPortsSameDT=off  OutDataTypeStr=boolean
  AND2 : Logic  AllPortsSameDT=off  OutDataTypeStr=boolean
  AND3 : Logic  Inputs=3  AllPortsSameDT=off  OutDataTypeStr=boolean
  AND4 : Logic  Operator=OR  AllPortsSameDT=off  OutDataTypeStr=boolean
  Relational Operator : RelationalOperator  Operator=<=  OutDataTypeStr=boolean  RndMeth=Nearest
  Relational Operator1 : RelationalOperator  Operator=<=  OutDataTypeStr=boolean  RndMeth=Nearest
  Unit Delay : UnitDelay  SampleTime=-1
  y : Outport
  wires:
  Relational Operator/1 -> AND1/1, AND2/1
  Relational Operator1/1 -> AND/1
  AND3/1 -> AND4/2
  AND4/1 -> Unit Delay/1, y/1
  AND/1 -> AND2/2, AND3/2
  on/1 -> Relational Operator/1
  In2/1 -> Relational Operator1/1, Relational Operator/2
  off/1 -> Relational Operator1/2
  AND2/1 -> AND4/1
  Unit Delay/1 -> AND3/3
  AND1/1 -> AND3/1

== system UXFD_Lib/Standard/Relation&Logic/SignalDelay3 ==
  note: S T E A D Y
  note: D E L A Y
  note: H O L D
  note: T R I G
  note: C O U N T E R
  In1 : Inport
  tdOn : Inport  Port=2
  tdOff : Inport  Port=3
  AND : Logic  Operator=OR  AllPortsSameDT=off  OutDataTypeStr=boolean
  AND1 : Logic  AllPortsSameDT=off  OutDataTypeStr=boolean
  Add : Sum  SaturateOnIntegerOverflow=on
  Constant : Constant  Value=0  OutDataTypeStr=Inherit: Inherit via back propagation
  Constant1 : Constant  Value=0  OutDataTypeStr=Inherit: Inherit via back propagation
  Relational Operator : RelationalOperator  Operator===  OutDataTypeStr=boolean  RndMeth=Nearest
  Relational Operator1 : RelationalOperator  Operator=>  OutDataTypeStr=boolean  RndMeth=Nearest
  Relational Operator2 : RelationalOperator  OutDataTypeStr=boolean  RndMeth=Nearest
  Relational Operator3 : RelationalOperator  Operator===  OutDataTypeStr=boolean  RndMeth=Nearest
  Switch : Switch  Criteria=u2 ~= 0  Threshold=0.5
  Switch1 : Switch  Criteria=u2 ~= 0  Threshold=0.5
  Unit Delay : UnitDelay  SampleTime=-1
  Unit Delay1 : UnitDelay  SampleTime=-1
  Unit Delay2 : UnitDelay  SampleTime=-1
  ts : DataStoreRead  DataStoreName=ts
  y : Outport
  wires:
  Relational Operator2/1 -> AND/2
  Relational Operator1/1 -> AND1/2
  AND1/1 -> AND/1
  AND/1 -> Unit Delay2/1, Relational Operator3/2
  Unit Delay2/1 -> AND1/1
  Constant1/1 -> Relational Operator1/2
  ts/1 -> Add/2
  Relational Operator3/1 -> y/1
  Switch1/1 -> Relational Operator2/2
  tdOff/1 -> Switch1/3
  Constant/1 -> Switch/3
  Switch/1 -> Unit Delay/1, Relational Operator2/1, Relational Operator1/1
  Unit Delay1/1 -> Relational Operator/1
  In1/1 -> Relational Operator3/1, Unit Delay1/1, Switch1/2, Relational Operator/2
  Add/1 -> Switch/1
  Unit Delay/1 -> Add/1
  Relational Operator/1 -> Switch/2
  tdOn/1 -> Switch1/1

== system UXFD_Lib/Standard/Relation&Logic/SignalTurnOffDelay ==
  note: True = 上面，cnt 清零
      | False = 下面 ，cnt 计数
  note: cnt 计数 < td,保持输出True
  u : Inport
  td : Inport  Port=2
  Add : Sum  SaturateOnIntegerOverflow=on
  Constant : Constant  Value=0
  Delay : Delay  DelayLength=1  InitialConditionSource=Input port  InitialCondition=0  InputProcessing=Inherited
      settings: InputPortMap=u0,p4
  Relational Operator : RelationalOperator  Operator=<=  OutDataTypeStr=boolean  RndMeth=Nearest
  Switch1 : Switch  Criteria=u2 ~= 0  Threshold=0.5
  ts : DataStoreRead  DataStoreName=ts
  y : Outport
  wires:
  Constant/1 -> Switch1/1
  Add/1 -> Switch1/3
  Relational Operator/1 -> y/1  "output"
  u/1 -> Switch1/2
  ts/1 -> Add/2
  Delay/1 -> Add/1
  Switch1/1 -> Delay/1, Relational Operator/1  "turnOffCnt"
  td/1 -> Delay/2, Relational Operator/2  "delay_td"

== system UXFD_Lib/Standard/Relation&Logic/SignalTurnOnDelay ==
  u : Inport
  td : Inport  Port=2
  Add : Sum  SaturateOnIntegerOverflow=on
  Constant : Constant  Value=0  OutDataTypeStr=Inherit: Inherit via back propagation
  Relational Operator : RelationalOperator  Operator=>  OutDataTypeStr=boolean  RndMeth=Nearest
  Switch1 : Switch  Criteria=u2 ~= 0  Threshold=0.5
  Unit Delay : UnitDelay  SampleTime=-1
  ts : DataStoreRead  DataStoreName=ts
  y : Outport
  wires:
  ts/1 -> Add/2
  Unit Delay/1 -> Add/1
  td/1 -> Relational Operator/2
  Switch1/1 -> Unit Delay/1, Relational Operator/1
  Add/1 -> Switch1/1
  Constant/1 -> Switch1/3
  u/1 -> Switch1/2
  Relational Operator/1 -> y/1

== system UXFD_Lib/Standard/Relation&Logic/SignalTurnOnOffDelay ==
  note: 1
  note: 0.01
  u : Inport
  td : Inport  Port=2
  Add : Sum  SaturateOnIntegerOverflow=on
  Delay : Delay  DelayLength=1  InitialConditionSource=Input port
      settings: InputPortMap=u0,p4
  Delay1 : Delay  DelayLength=1  InitialConditionSource=Input port
      settings: InputPortMap=u0,p4
  Relational Operator : RelationalOperator  Operator===  OutDataTypeStr=boolean  RndMeth=Nearest
  Relational Operator1 : RelationalOperator  Operator=>  OutDataTypeStr=boolean  RndMeth=Nearest
  Switch : Switch  Criteria=u2 ~= 0  Threshold=0.5  OutDataTypeStr=Inherit: Inherit via back propagation
  Switch1 : Switch  Criteria=u2 ~= 0  Threshold=0.5
  Unit Delay1 : UnitDelay  SampleTime=-1
  ts : DataStoreRead  DataStoreName=ts
  y : Outport
  wires:
  Switch1/1 -> Delay1/1, y/1
  Delay1/1 -> Switch1/3
  Relational Operator1/1 -> Switch1/2
  Relational Operator/1 -> Switch/2
  Add/1 -> Switch/1
  Switch/1 -> Unit Delay1/1, Relational Operator1/1
  td/1 -> Relational Operator1/2
  Unit Delay1/1 -> Add/1
  ts/1 -> Switch/3, Add/2
  u/1 -> Delay/1, Delay/2, Delay1/2, Switch1/1, Relational Operator/1
  Delay/1 -> Relational Operator/2

== system UXFD_Lib/Standard/Relation&Logic/xbackground1 ==

== system UXFD_Lib/Standard/Relation&Logic/xbackground2 ==

== system UXFD_Lib/Standard/Relation&Logic/xbackground3 ==

== system UXFD_Lib/Standard/Relation&Logic/xbackground4 ==

== system UXFD_Lib/Standard/Relation&Logic/xbackground5 ==

== system UXFD_Lib/Standard/Relation&Logic/xbackground6 ==

== system UXFD_Lib/Standard/Relation&Logic/xbackground7 ==

== system UXFD_Lib/Standard/Relation&Logic/xbackground8 ==

== system UXFD_Lib/Standard/Relation&Logic/xbackground9 ==

== system UXFD_Lib/Standard/Signals and systems/ESubsystem ==
  Enable_Name : EnablePort

== system UXFD_Lib/Standard/Signals and systems/ETSubsystem ==
  Enable_Name : EnablePort
  Trigger_Name : TriggerPort  VariantControl=Variant

== system UXFD_Lib/Standard/Signals and systems/Function-Call Subsystem ==
  In1 : Inport
  function : TriggerPort  TriggerType=function-call  VariantControl=Variant
  Out1 : Outport
  wires:
  In1/1 -> Out1/1

== system UXFD_Lib/Standard/Signals and systems/Model Header ==

== system UXFD_Lib/Standard/Signals and systems/RenameSignal ==
  Inport : Inport
  y : Outport
  wires:
  Inport/1 -> y/1

== system UXFD_Lib/Standard/Signals and systems/Subsystem ==
  In1 : Inport
  Out1 : Outport
  wires:
  In1/1 -> Out1/1

== system UXFD_Lib/Standard/Signals and systems/TSubsystem ==
  Trigger_Name : TriggerPort  VariantControl=Variant

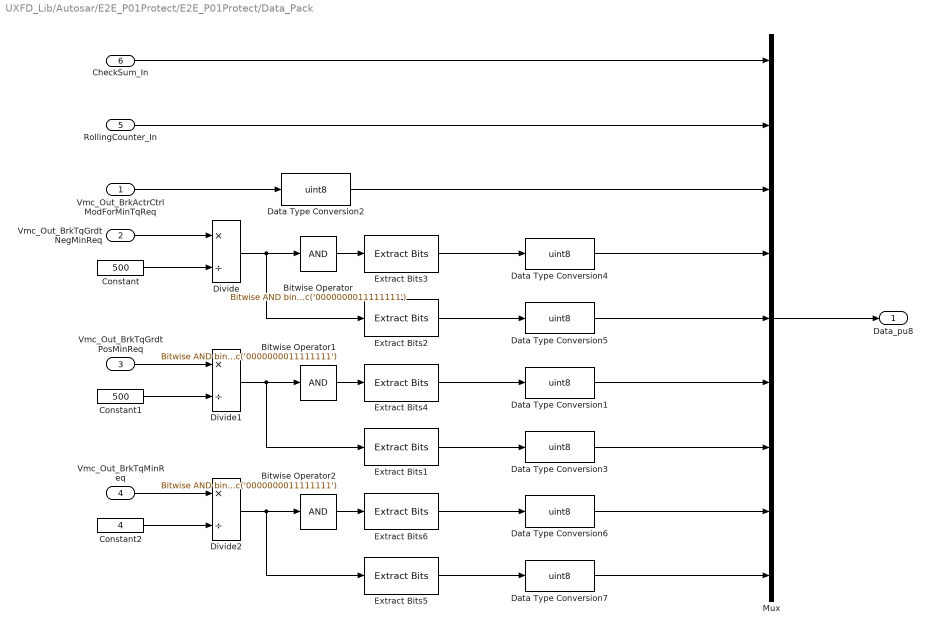
== system UXFD_Lib/Autosar/E2E_P01Protect/E2E_P01Protect/Data_Pack ==
  Vmc_Out_BrkActrCtrlModForMinTqReq : Inport
  Vmc_Out_BrkTqGrdtNegMinReq : Inport  Port=2
  Vmc_Out_BrkTqGrdtPosMinReq : Inport  Port=3
  Vmc_Out_BrkTqMinReq : Inport  Port=4
  RollingCounter_In : Inport  Port=5
  CheckSum_In : Inport  Port=6
  Bitwise Operator : simulink/Logic and Bit Operations/Bitwise Operator  logicop=AND  UseBitMask=on  BitMask=bin2dec('0000000011111111')  BitMaskRealWorld=Stored Integer
  Bitwise Operator1 : simulink/Logic and Bit Operations/Bitwise Operator  logicop=AND  UseBitMask=on  BitMask=bin2dec('0000000011111111')  BitMaskRealWorld=Stored Integer
  Bitwise Operator2 : simulink/Logic and Bit Operations/Bitwise Operator  logicop=AND  UseBitMask=on  BitMask=bin2dec('0000000011111111')  BitMaskRealWorld=Stored Integer
  Constant : Constant  Value=500  OutDataTypeStr=uint16
      settings: CopyFcn=set_param(gcbh,'ShowName','off');
  Constant1 : Constant  Value=500  OutDataTypeStr=uint16
      settings: CopyFcn=set_param(gcbh,'ShowName','off');
  Constant2 : Constant  Value=4  OutDataTypeStr=uint8
      settings: CopyFcn=set_param(gcbh,'ShowName','off');
  Data Type Conversion{1..7} (7 alike) : DataTypeConversion  OutDataTypeStr=uint8
  Divide : Product  Inputs=*/  OutDataTypeStr=uint16
  Divide1 : Product  Inputs=*/  OutDataTypeStr=uint16
  Divide2 : Product  Inputs=*/  OutDataTypeStr=uint16
  Extract Bits1 : simulink/Logic and Bit Operations/Extract Bits  bitsToExtract=Upper half  numBits=8  bitIdxRange=[0 7]  outScalingMode=Treat bit field as an integer
  Extract Bits2 : simulink/Logic and Bit Operations/Extract Bits  bitsToExtract=Upper half  numBits=8  bitIdxRange=[0 7]  outScalingMode=Treat bit field as an integer
  Extract Bits3 : simulink/Logic and Bit Operations/Extract Bits  bitsToExtract=Lower half  numBits=8  bitIdxRange=[0 7]  outScalingMode=Treat bit field as an integer
  Extract Bits4 : simulink/Logic and Bit Operations/Extract Bits  bitsToExtract=Lower half  numBits=8  bitIdxRange=[0 7]  outScalingMode=Treat bit field as an integer
  Extract Bits5 : simulink/Logic and Bit Operations/Extract Bits  bitsToExtract=Upper half  numBits=8  bitIdxRange=[0 7]  outScalingMode=Treat bit field as an integer
  Extract Bits6 : simulink/Logic and Bit Operations/Extract Bits  bitsToExtract=Lower half  numBits=8  bitIdxRange=[0 7]  outScalingMode=Treat bit field as an integer
  Mux : Mux  Inputs=9
  Data_pu8 : Outport
  wires:
  Mux/1 -> Data_pu8/1
  Vmc_Out_BrkActrCtrlModForMinTqReq/1 -> Data Type Conversion2/1
  Extract Bits3/1 -> Data Type Conversion4/1
  Constant/1 -> Divide/2
  Bitwise Operator/1 -> Extract Bits3/1
  Extract Bits2/1 -> Data Type Conversion5/1
  Divide/1 -> Extract Bits2/1, Bitwise Operator/1
  Vmc_Out_BrkTqGrdtNegMinReq/1 -> Divide/1
  Extract Bits4/1 -> Data Type Conversion1/1
  Constant1/1 -> Divide1/2
  Bitwise Operator1/1 -> Extract Bits4/1
  Extract Bits1/1 -> Data Type Conversion3/1
  Divide1/1 -> Extract Bits1/1, Bitwise Operator1/1
  Vmc_Out_BrkTqGrdtPosMinReq/1 -> Divide1/1
  Extract Bits6/1 -> Data Type Conversion6/1
  Constant2/1 -> Divide2/2
  Bitwise Operator2/1 -> Extract Bits6/1
  Extract Bits5/1 -> Data Type Conversion7/1
  Divide2/1 -> Extract Bits5/1, Bitwise Operator2/1
  Vmc_Out_BrkTqMinReq/1 -> Divide2/1
  RollingCounter_In/1 -> Mux/2
  CheckSum_In/1 -> Mux/1
  Data Type Conversion2/1 -> Mux/3
  Data Type Conversion4/1 -> Mux/4
  Data Type Conversion5/1 -> Mux/5
  Data Type Conversion1/1 -> Mux/6
  Data Type Conversion3/1 -> Mux/7
  Data Type Conversion6/1 -> Mux/8
  Data Type Conversion7/1 -> Mux/9

== system UXFD_Lib/Autosar/E2E_P01Protect/E2E_P01Protect/E2E_Config ==
  DataLength : Inport
  DataID : Inport  Port=2
  BusCreator : BusCreator  Inputs=6  OutDataTypeStr=Bus: E2E_P01ConfigType  NonVirtualBus=on
      settings: CopyFcn=set_param(gcbh,'ShowName','off');  InheritFromInputs=off
  CRCOffset : Constant  Value=0  OutDataTypeStr=uint16
  CounterOffset : Constant  Value=8  OutDataTypeStr=uint16
  DataIDMode : simulink/Sources/Enumerated Constant  OutDataTypeStr=Enum: E2E_P01DataIDMode  Value=E2E_P01DataIDMode.E2E_P01_DATAID_BOTH  SampleTime=inf
  MaxDeltaCounterInit : Constant  Value=14  OutDataTypeStr=uint8
  E2E_P01_Config : Outport
  wires:
  DataID/1 -> BusCreator/2
  CounterOffset/1 -> BusCreator/6
  MaxDeltaCounterInit/1 -> BusCreator/4
  BusCreator/1 -> E2E_P01_Config/1
  DataIDMode/1 -> BusCreator/3
  DataLength/1 -> BusCreator/1
  CRCOffset/1 -> BusCreator/5

== system UXFD_Lib/Autosar/E2E_P01Protect/E2E_P01Protect/E2E_P01Protect_S ==
  ConfigType : Inport
  SenderStateType : Inport  Port=2
  Data_pu8 : Inport  Port=3
  S-Function : S-Function  FunctionName=E2E_P01Protect_S  SFunctionDeploymentMode=off  EnableBusSupport=off
  Std_ReturnType : Outport
  wires:
  S-Function/1 -> Std_ReturnType/1
  Data_pu8/1 -> S-Function/3
  ConfigType/1 -> S-Function/1
  SenderStateType/1 -> S-Function/2

== system UXFD_Lib/Autosar/E2E_P01_Check/E2E_Check/E2E_Check ==
  Status : Inport
  DataLength : Inport  Port=2
  DataID : Inport  Port=3
  AccrPedlNotCmpl_IsUpdated : Inport  Port=4
  CheckSum : Inport  Port=5
  RollingCounter : Inport  Port=6
  AccrPedlNotCmpl_Psd : Inport  Port=7
  AccrPedlNotCmpl_PsdSts : Inport  Port=8
  Data_ID_218 : Subsystem
  E2E_Config_ID_218 : Subsystem
  E2E_P01Check_S : Subsystem
      mask Display:
      | disp('E2E_P01Check');
      | port_label('input',1,'ConfigType');
      | port_label('input',2,'ReceiverStateType');
      | port_label('input',3,'Data_pu8');
      | port_label('output',1,'Std_ReturnType');
  E2E_P01ReceiverID_218 : Subsystem
  E2E_P01Check_ReturnType : Outport
  E2E_P01ReceiverStatus : Outport  Port=2
  wires:
  RollingCounter/1 -> Data_ID_218/2(RollingCounter)
  CheckSum/1 -> Data_ID_218/1(CheckSum)
  Data_ID_218/1(Data_pu8) -> E2E_P01Check_S/3(Data_pu8)
  E2E_P01Check_S/1(Std_ReturnType) -> E2E_P01Check_ReturnType/1
  E2E_Config_ID_218/1(E2E_Config_ID_218) -> E2E_P01Check_S/1(ConfigType)
  AccrPedlNotCmpl_IsUpdated/1 -> E2E_P01ReceiverID_218/1(AccrPedlNotCmpl_IsUpdated)
  DataLength/1 -> E2E_Config_ID_218/1(DataLength)
  E2E_P01ReceiverID_218/1(E2E_P01ReceiverState) -> E2E_P01ReceiverStatus/1, E2E_P01Check_S/2(ReceiverStateType)
  DataID/1 -> E2E_Config_ID_218/2(DataID)
  Status/1 -> E2E_P01ReceiverID_218/2(Status)
  AccrPedlNotCmpl_Psd/1 -> Data_ID_218/3(AccrPedlNotCmpl_Psd)
  AccrPedlNotCmpl_PsdSts/1 -> Data_ID_218/4(AccrPedlNotCmpl_PsdSts)

== system UXFD_Lib/Custom/CAN/CanHex2Signed/condtion ==
  note: 判断条件:2^(n-1)-1
  note: 模：2^n
  bitL : Inport
  Add : Sum  Inputs=+-
      settings: CopyFcn=set_param(gcbh,'ShowName','off');
  Add1 : Sum  Inputs=+-
      settings: CopyFcn=set_param(gcbh,'ShowName','off');
  Constant : Constant  Value=2  OutDataTypeStr=single
      settings: CopyFcn=set_param(gcbh,'ShowName','off');
  Constant1 : Constant  OutDataTypeStr=single
      settings: CopyFcn=set_param(gcbh,'ShowName','off');
  Constant3 : Constant  OutDataTypeStr=uint8
      settings: CopyFcn=set_param(gcbh,'ShowName','off');
  Constant4 : Constant  Value=2  OutDataTypeStr=single
      settings: CopyFcn=set_param(gcbh,'ShowName','off');
  Gain : Gain  OutDataTypeStr=uint32
      settings: CopyFcn=set_param(gcbh,'ShowName','off');
  Math Function : Math  Operator=pow  OutputSignalType=real  SaturateOnIntegerOverflow=on
  Math Function1 : Math  Operator=pow  OutputSignalType=real  SaturateOnIntegerOverflow=on
  cond : Outport
  2^n : Outport  Port=2
  wires:
  Add/1 -> cond/1
  Gain/1 -> Add/1
  Constant4/1 -> Math Function1/1
  Add1/1 -> Math Function1/2
  Constant1/1 -> Add1/2
  Constant/1 -> Math Function/1
  Math Function/1 -> 2^n/1
  Math Function1/1 -> Gain/1
  Constant3/1 -> Add/2
  bitL/1 -> Math Function/2, Add1/1
